simulink model "three_phase_dab"  (R2025b)
settings: Solver=ode23tb  StartTime=0.0  StopTime=simlength  FixedStep=tc  MaxStep=tc
values from neighbouring files (symbols this model uses):
  Idc_FS = max(Idab1_dc_nom,Idab2_dc_nom) * margin_factor    [init_model.m]
  tc = ts_dab/100    (= 4.16666666667e-07)    [init_model.m]
  Vdab2_dc_nom = 1500    [init_model.m]
  Vdc_FS = max(Vdab1_dc_nom,Vdab2_dc_nom) * margin_factor    [init_model.m]
libraries: fl_lib x27, nesl_utility x23, discrete_time_low_pass_filter x6, single_phase_transformer x3, single_phase_transformer_lib x3, litium_ion_battery x2, pi_ctrl x2, three_phase_inverter_ideal_switch_based_model x2, three_phase_inverter_mosfet_based_with_thermal_model x2, three_phase_dab_modulator x1
(part 1 of 2)
settings Model: SimulationMode=accelerator  Creator=LTNBDA  LastModifiedBy=dbagn
settings SolverCC: ZeroCrossControl=EnableAll  ZeroCrossAlgorithm=Adaptive  AlgebraicLoopSolver=TrustRegion  SolverResetMethod=Robust  AutoInsertRateTranBlk=on
settings DataIOCC: LimitDataPoints=on  MaxDataPoints=1  SaveFormat=Array  SignalLoggingSaveFormat=ModelDataLogs  SaveOutput=off  SignalLogging=off  DSMLogging=off  SaveTime=off  ReturnWorkspaceOutputs=off
settings OptimizationCC: ExpressionDepthLimit=2147483647.0  InitFltsAndDblsToZero=on  EfficientMapNaN2IntZero=off  LifeSpan=inf
settings DebuggingCC: SaveWithParameterizedLinksMsg=none  UnderspecifiedInitializationDetection=Classic  MergeDetectMultiDrivingBlocksExec=none  SignalResolutionControl=TryResolveAllWithWarning  SolverPrmCheckMsg=warning  MultiTaskDSMMsg=warning  MultiTaskCondExecSysMsg=none  MultiTaskRateTransMsg=warning  FcnCallInpInsideContextMsg=warning  StateNameClashWarn=warning  SFUnexpectedBacktrackingDiag=warning  SFNoUnconditionalDefaultTransitionDiag=warning  ArithmeticOperatorsInVariantConditions=warning
settings HardwareCC: ProdBitPerLong=64.0  ProdLargestAtomicFloat=None  ProdIntDivRoundTo=Undefined  ProdEndianess=Unspecified  ProdHWDeviceType=Generic->64-bit Embedded Processor (LP64)  TargetBitPerPointer=64.0  TargetBitPerSizeT=64.0  TargetBitPerPtrDiffT=64.0  TargetLongLongMode=on  TargetIntDivRoundTo=Zero  TargetEndianess=LittleEndian  TargetWordSize=64.0  TargetHWDeviceType=MATLAB Host  ProdEqTarget=off
settings ModelReferenceCC: EnableRefExpFcnMdlSchedulingChecks=on  PropagateSignalLabelsOutOfModel=off
settings SFSimCC: SimUseLocalCustomCode=off  CustomCodeUndefinedFunction=UseInterfaceOnly
settings RTWCC: RTWUseLocalCustomCode=off  GPUComputeCapability=3.5
settings CodeAppCC: MaxIdLength=128.0  StateflowObjectComments=on
settings GRTTargetCC: TargetLangStandard=C89/C90 (ANSI)  CombineOutputUpdateFcns=off  GRTInterface=on
settings ConfigComp: CovMetricSettings=dw  CovSaveCumulativeToWorkspaceVar=on  CovSaveSingleToWorkspaceVar=on  CovExternalEMLEnable=off
settings SimscapeCC: SimscapeNormalizeSystem=off

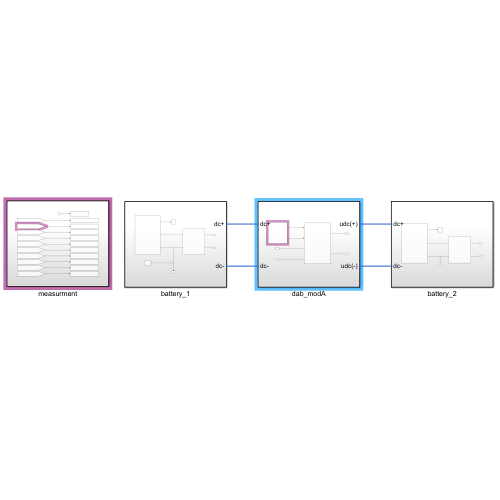
[thumbnail: Simulink's stored preview of the top-level diagram]
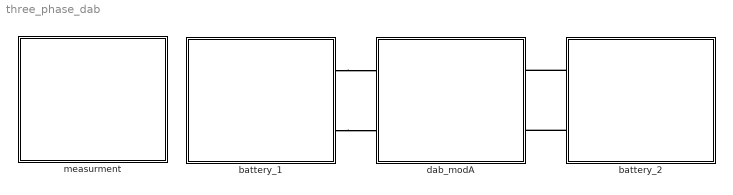
== system three_phase_dab ==
  battery_1 : Subsystem
  battery_2 : Subsystem
  dab_modA : Subsystem
  measurment : Subsystem
  connections:
  battery_2/RConn2 -- dab_modA/RConn2
  battery_2/RConn1 -- dab_modA/RConn1
  battery_1/RConn1 -- dab_modA/LConn1
  battery_1/RConn2 -- dab_modA/LConn2

== system three_phase_dab/battery_1 ==
  Electrical Reference1 : fl_lib/Electrical/Electrical Elements/Electrical Reference
  Solver Configuration : nesl_utility/Solver Configuration  PhysicalDomain=network_engine_domain  SubClassName=solver  LeftPortType=input  RightPortType=generic  Tones=[]  Harmonics=[]  SimulateNoise=off  Profile=off  UseLocalSampling=off  EnableSwitchedLinearOptims=on  FrequencyDomain=off  UseCCode=off  RelTol=0.001  AbsTol=0.001  MinStep=1e-09  ToWorkspace=off  RevertToSquareIcSolve=off  NumHomotopyIterations=100  PhasorMode=off  PhasorModeNumHarmonics=1  ConsistencySolver=NEWTON_FTOL  IndexReductionMethod=DerivativeReplacement  DoDC=off  ResidualTolerance=1e-09  ConsistencyTolSource=GLOBAL  ConsistencyAbsTol=0.001  ConsistencyRelTol=0.001  ConsistencyTolFactor=0.001  UseLocalSolver=on  LocalSolverChoice=NE_BACKWARD_EULER_ADVANCER  ResolveIndetEquations=on  FunctionEvalNumThread=1  LocalSolverSampleTime=tc  DoFixedCost=on  MaxNonlinIter=3  MaxModeIter=2  ComputeImpulses=off  ImpulseIterations=2  LinearAlgebra=auto  LinearAlgebraNumThread=0  EquationFormulation=NE_TIME_EF  DelaysMemoryBudget=1024  AutomaticFiltering=on  FilteringTimeConstant=0.001  PartitionStorageMethod=AS_NEEDED  PartitionMemoryBudget=1024  PartitionMethod=ROBUST  MultibodyUseLocalSolver=off  MultibodyLocalSolverChoice=ODE1  MultibodyLocalSolverSampleTime=0.001
  litium ion battery 1 : Scope
      settings: ActiveDisplayYMinimum=1095.5241232297076  ActiveDisplayYMaximum=1432.6160946881369  DataLoggingVariableName=ScopeData3
  litium_ion_battery : litium_ion_battery/litium_ion_battery  Q=50  number_of_cells=346  E_1=-1.031  E0=3.485  E1=0  E2=0  E3=0  Elog=-0.05  R0=0.035  R1=0.035  C1=0.5  M=125  alpha=35  soc_init=0.85  ts_battery=ts_battery  q1Kalman=q1Kalman  q2Kalman=q2Kalman  q3Kalman=q3Kalman  rKalman=rKalman  tc=tc
  single_phase_ui_measure : Subsystem
  dc+ : PMIOPort  Side=Right
  dc- : PMIOPort  Port=2  Side=Right
  wires:
  litium_ion_battery/1 -> litium ion battery 1/1
  connections:
  litium_ion_battery/RConn2 -- single_phase_ui_measure/LConn2 -- Electrical Reference1/LConn1 -- Solver Configuration/RConn1
  single_phase_ui_measure/RConn1 -- dc+/RConn1
  single_phase_ui_measure/LConn1 -- litium_ion_battery/RConn1
  dc-/RConn1 -- single_phase_ui_measure/RConn2

== system three_phase_dab/battery_2 ==
  Electrical Reference1 : fl_lib/Electrical/Electrical Elements/Electrical Reference
  litium ion battery 2 : Scope
      settings: ActiveDisplayYMinimum=-748.38980710578858  ActiveDisplayYMaximum=3166.4304287109808  DataLoggingVariableName=ScopeData3
  litium_ion_battery : litium_ion_battery/litium_ion_battery  Q=50  number_of_cells=346  E_1=-1.031  E0=3.485  E1=0  E2=0  E3=0  Elog=-0.05  R0=0.035  R1=0.035  C1=0.5  M=125  alpha=35  soc_init=0.85  ts_battery=ts_battery  q1Kalman=q1Kalman  q2Kalman=q2Kalman  q3Kalman=q3Kalman  rKalman=rKalman  tc=tc
  single_phase_ui_measure : Subsystem
  dc+ : PMIOPort  Side=Right
  dc- : PMIOPort  Port=2  Side=Right
  wires:
  litium_ion_battery/1 -> litium ion battery 2/1
  connections:
  dc-/RConn1 -- single_phase_ui_measure/RConn2
  single_phase_ui_measure/LConn1 -- litium_ion_battery/RConn1
  single_phase_ui_measure/RConn1 -- dc+/RConn1
  Electrical Reference1/LConn1 -- single_phase_ui_measure/LConn2 -- litium_ion_battery/RConn2

== system three_phase_dab/dab_modA ==
  dab_ctrl : Subsystem
  dcdc_with_galvanic_isolation : Subsystem
  udc(+) : PMIOPort  Side=Right
  udc(-) : PMIOPort  Port=2  Side=Right
  dc+ : PMIOPort  Port=3  Side=Left
  dc- : PMIOPort  Port=4  Side=Left
  wires:
  dab_ctrl/2(gate_commands_2) -> dcdc_with_galvanic_isolation/2(gate_commands_1)
  dab_ctrl/1(gate_commands_1) -> dcdc_with_galvanic_isolation/1(gate_commands_2)
  connections:
  udc(+)/RConn1 -- dcdc_with_galvanic_isolation/RConn1
  udc(-)/RConn1 -- dcdc_with_galvanic_isolation/RConn2
  dc-/RConn1 -- dcdc_with_galvanic_isolation/LConn2
  dc+/RConn1 -- dcdc_with_galvanic_isolation/LConn1

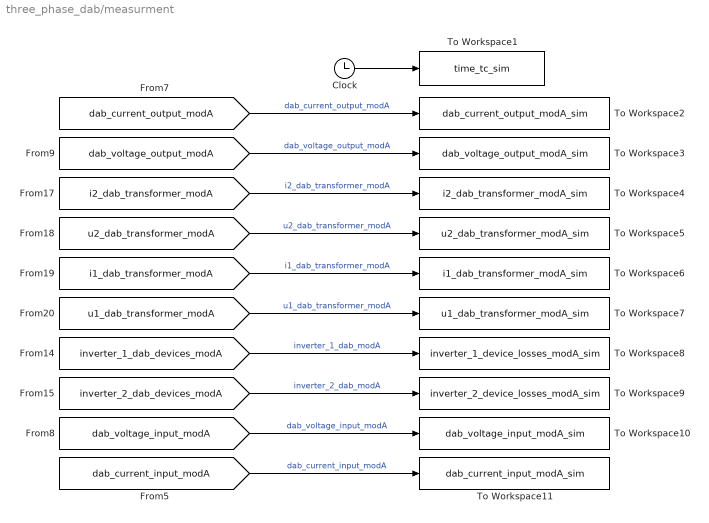
== system three_phase_dab/measurment ==
  Clock : Clock
  To Workspace1 : ToWorkspace  VariableName=time_tc_sim  SampleTime=tc
      settings: MaxDataPoints=Nc
  To Workspace10 : ToWorkspace  VariableName=dab_voltage_input_modA_sim  SampleTime=tc
      settings: MaxDataPoints=Nc
  To Workspace11 : ToWorkspace  VariableName=dab_current_input_modA_sim  SampleTime=tc
      settings: MaxDataPoints=Nc
  To Workspace2 : ToWorkspace  VariableName=dab_current_output_modA_sim  SampleTime=tc
      settings: MaxDataPoints=Nc
  To Workspace3 : ToWorkspace  VariableName=dab_voltage_output_modA_sim  SampleTime=tc
      settings: MaxDataPoints=Nc
  To Workspace4 : ToWorkspace  VariableName=i2_dab_transformer_modA_sim  SampleTime=tc
      settings: MaxDataPoints=Nc
  To Workspace5 : ToWorkspace  VariableName=u2_dab_transformer_modA_sim  SampleTime=tc
      settings: MaxDataPoints=Nc
  To Workspace6 : ToWorkspace  VariableName=i1_dab_transformer_modA_sim  SampleTime=tc
      settings: MaxDataPoints=Nc
  To Workspace7 : ToWorkspace  VariableName=u1_dab_transformer_modA_sim  SampleTime=tc
      settings: MaxDataPoints=Nc
  To Workspace8 : ToWorkspace  VariableName=inverter_1_device_losses_modA_sim  SampleTime=tc
      settings: MaxDataPoints=Nc
  To Workspace9 : ToWorkspace  VariableName=inverter_2_device_losses_modA_sim  SampleTime=tc
      settings: MaxDataPoints=Nc
  wires:
  Clock/1 -> To Workspace1/1
  [dab_current_output_modA] -> To Workspace2/1  "dab_current_output_modA"
  [dab_voltage_output_modA] -> To Workspace3/1  "dab_voltage_output_modA"
  [i2_dab_transformer_modA] -> To Workspace4/1  "i2_dab_transformer_modA"
  [u1_dab_transformer_modA] -> To Workspace7/1  "u1_dab_transformer_modA"
  [i1_dab_transformer_modA] -> To Workspace6/1  "i1_dab_transformer_modA"
  [u2_dab_transformer_modA] -> To Workspace5/1  "u2_dab_transformer_modA"
  [inverter_1_dab_devices_modA] -> To Workspace8/1  "inverter_1_dab_modA"
  [inverter_2_dab_devices_modA] -> To Workspace9/1  "inverter_2_dab_modA"
  [dab_voltage_input_modA] -> To Workspace10/1  "dab_voltage_input_modA"
  [dab_current_input_modA] -> To Workspace11/1  "dab_current_input_modA"

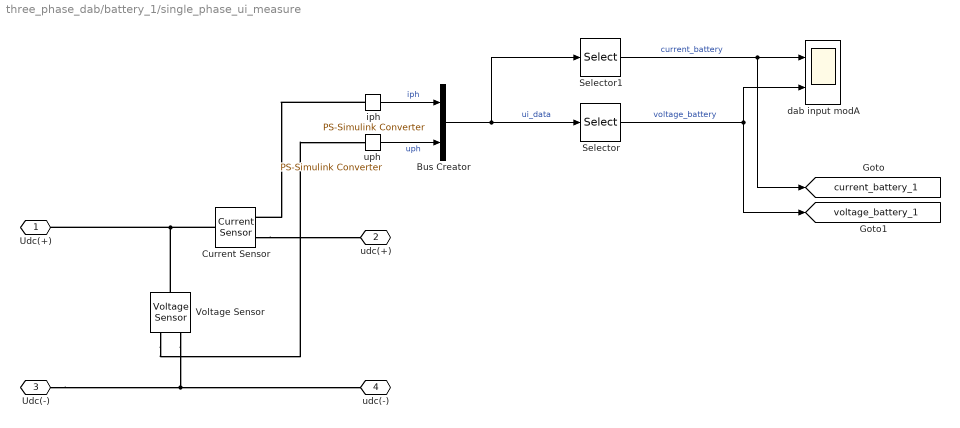
== system three_phase_dab/battery_1/single_phase_ui_measure ==
  Bus Creator : BusCreator  Inputs=2
  Current Sensor : fl_lib/Electrical/Electrical Sensors/Current Sensor
  Selector : Selector  InputPortWidth=2  IndexOptions=Index vector (dialog)  Indices=2  OutputSizes=1
  Selector1 : Selector  InputPortWidth=2  IndexOptions=Index vector (dialog)  Indices=1  OutputSizes=1
  Voltage Sensor : fl_lib/Electrical/Electrical Sensors/Voltage Sensor
  dab input modA : Scope  NumInputPorts=2
      settings: SampleTime=tc  ActiveDisplayYMinimum=-4428.9106738971032  ActiveDisplayYMaximum=4853.7975894934307  DataLoggingVariableName=ScopeData2
  iph : nesl_utility/PS-Simulink Converter  PhysicalDomain=network_engine_domain  SubClassName=ps_output  LeftPortType=input  RightPortType=output  PseudoPeriodic=off  Frequencies=[]  VectorFormat=1-D array  Unit=A  AffineConversion=off
  uph : nesl_utility/PS-Simulink Converter  PhysicalDomain=network_engine_domain  SubClassName=ps_output  LeftPortType=input  RightPortType=output  PseudoPeriodic=off  Frequencies=[]  VectorFormat=1-D array  Unit=V  AffineConversion=off
  Udc(+) : PMIOPort  Side=Left
  udc(+) : PMIOPort  Port=2  Side=Right
  Udc(-) : PMIOPort  Port=3  Side=Left
  udc(-) : PMIOPort  Port=4  Side=Right
  tag scope: current_battery_1=global, voltage_battery_1=global
  wires:
  Bus Creator/1 -> Selector/1, Selector1/1  "ui_data"
  iph/1 -> Bus Creator/1  "iph"
  uph/1 -> Bus Creator/2  "uph"
  Selector1/1 -> [current_battery_1], dab input modA/1  "current_battery"
  Selector/1 -> dab input modA/2, [voltage_battery_1]  "voltage_battery"
  connections:
  iph/LConn1 -- Current Sensor/RConn1
  Voltage Sensor/LConn1 -- Current Sensor/LConn1 -- Udc(+)/RConn1
  Current Sensor/RConn2 -- udc(+)/RConn1
  Voltage Sensor/RConn1 -- uph/LConn1
  Voltage Sensor/RConn2 -- Udc(-)/RConn1 -- udc(-)/RConn1

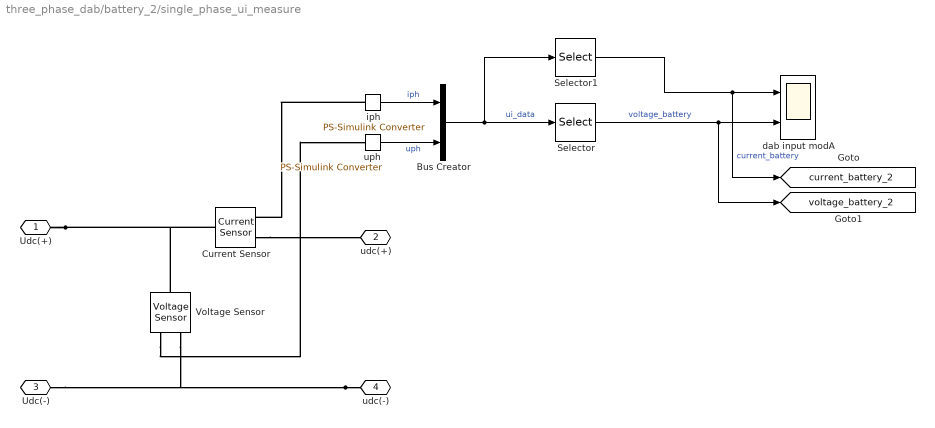
== system three_phase_dab/battery_2/single_phase_ui_measure ==
  Bus Creator : BusCreator  Inputs=2
  Current Sensor : fl_lib/Electrical/Electrical Sensors/Current Sensor
  Selector : Selector  InputPortWidth=2  IndexOptions=Index vector (dialog)  Indices=2  OutputSizes=1
  Selector1 : Selector  InputPortWidth=2  IndexOptions=Index vector (dialog)  Indices=1  OutputSizes=1
  Voltage Sensor : fl_lib/Electrical/Electrical Sensors/Voltage Sensor
  dab input modA : Scope  NumInputPorts=2
      settings: SampleTime=tc  ActiveDisplayYMinimum=-363.9315036867377  ActiveDisplayYMaximum=456.02820990604641  DataLoggingVariableName=ScopeData2
  iph : nesl_utility/PS-Simulink Converter  PhysicalDomain=network_engine_domain  SubClassName=ps_output  LeftPortType=input  RightPortType=output  PseudoPeriodic=off  Frequencies=[]  VectorFormat=1-D array  Unit=A  AffineConversion=off
  uph : nesl_utility/PS-Simulink Converter  PhysicalDomain=network_engine_domain  SubClassName=ps_output  LeftPortType=input  RightPortType=output  PseudoPeriodic=off  Frequencies=[]  VectorFormat=1-D array  Unit=V  AffineConversion=off
  Udc(+) : PMIOPort  Side=Left
  udc(+) : PMIOPort  Port=2  Side=Right
  Udc(-) : PMIOPort  Port=3  Side=Left
  udc(-) : PMIOPort  Port=4  Side=Right
  tag scope: current_battery_2=global, voltage_battery_2=global
  wires:
  Selector/1 -> [voltage_battery_2], dab input modA/2  "voltage_battery"
  Selector1/1 -> dab input modA/1, [current_battery_2]  "current_battery"
  uph/1 -> Bus Creator/2  "uph"
  iph/1 -> Bus Creator/1  "iph"
  Bus Creator/1 -> Selector1/1, Selector/1  "ui_data"
  connections:
  udc(-)/RConn1 -- Udc(-)/RConn1 -- Voltage Sensor/RConn2
  Voltage Sensor/RConn1 -- uph/LConn1
  Current Sensor/RConn2 -- udc(+)/RConn1
  Udc(+)/RConn1 -- Current Sensor/LConn1 -- Voltage Sensor/LConn1
  iph/LConn1 -- Current Sensor/RConn1

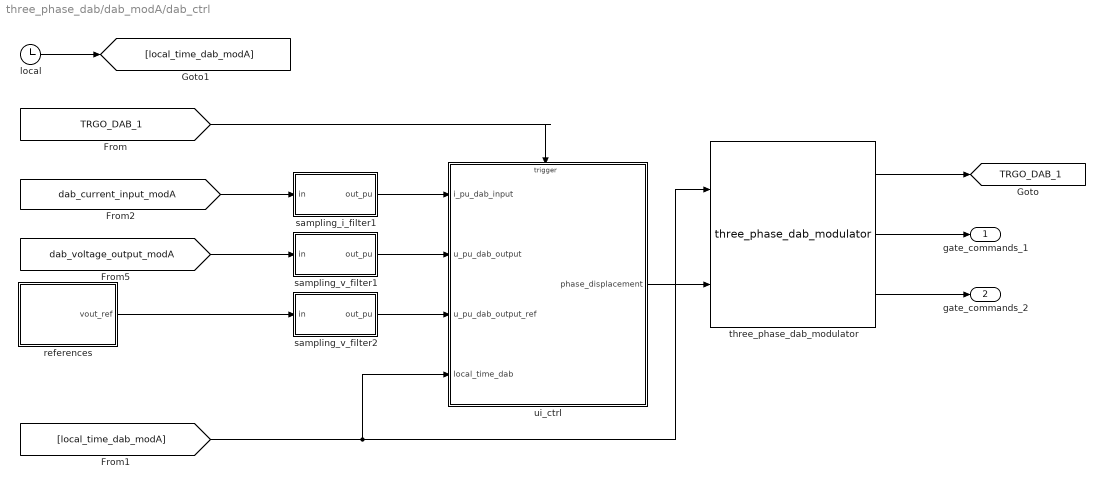
== system three_phase_dab/dab_modA/dab_ctrl ==
  local : Clock
  references : Subsystem
  sampling_i_filter1 : Subsystem
  sampling_v_filter1 : Subsystem
  sampling_v_filter2 : Subsystem
  three_phase_dab_modulator : three_phase_dab_modulator/three_phase_dab_modulator  fpwm=fPWM_DAB  tc=tc
  ui_ctrl : Subsystem
  gate_commands_1 : Outport
  gate_commands_2 : Outport  Port=2
  tag scope: TRGO_DAB_1=global
  wires:
  [dab_voltage_output_modA] -> sampling_v_filter1/1(in)
  [dab_current_input_modA] -> sampling_i_filter1/1(in)
  sampling_i_filter1/1(out_pu) -> ui_ctrl/1(i_pu_dab_input)
  sampling_v_filter1/1(out_pu) -> ui_ctrl/2(u_pu_dab_output)
  sampling_v_filter2/1(out_pu) -> ui_ctrl/3(u_pu_dab_output_ref)
  references/1(vout_ref) -> sampling_v_filter2/1(in)
  three_phase_dab_modulator/1 -> [TRGO_DAB_1]
  [TRGO_DAB_1] -> ui_ctrl/Trigger
  ui_ctrl/1(phase_displacement) -> three_phase_dab_modulator/2
  three_phase_dab_modulator/2 -> gate_commands_1/1
  three_phase_dab_modulator/3 -> gate_commands_2/1
  local/1 -> [local_time_dab_modA]
  [local_time_dab_modA] -> three_phase_dab_modulator/1, ui_ctrl/4(local_time_dab)

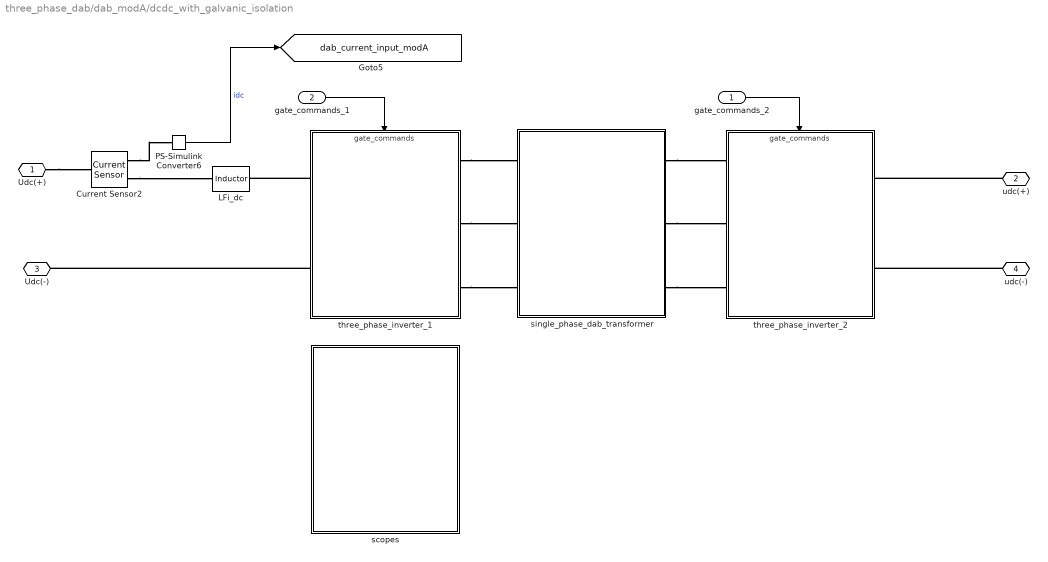
== system three_phase_dab/dab_modA/dcdc_with_galvanic_isolation ==
  gate_commands_2 : Inport
  gate_commands_1 : Inport  Port=2
  Current Sensor2 : fl_lib/Electrical/Electrical Sensors/Current Sensor
  LFi_dc : fl_lib/Electrical/Electrical Elements/Inductor  l=LFi_dc H  r=RLFi_dc Ohm  g=1e-9 1/Ohm  i_specify=off  i_priority=None  i=0 A  i_nominal_specify=off  i_nominal_value=1  i_nominal_unit=A  v_specify=off  v_priority=None  v=0 V  v_nominal_specify=off  v_nominal_value=1  v_nominal_unit=V  i_L_specify=off  i_L_priority=High  i_L=0 A  i_L_nominal_specify=off  i_L_nominal_value=1  i_L_nominal_unit=A
  PS-Simulink Converter6 : nesl_utility/PS-Simulink Converter  PhysicalDomain=network_engine_domain  SubClassName=ps_output  LeftPortType=input  RightPortType=output  PseudoPeriodic=off  Frequencies=[]  VectorFormat=1-D array  Unit=A  AffineConversion=on
  scopes : Subsystem
  single_phase_dab_transformer : Subsystem
  three_phase_inverter_1 : Subsystem
      settings: PortSchema="{\"entries\":[{\"content\":{\"sides\":[{\"content\":{\"connectorIds\":[\"LConn1\",\"LConn2\",\"LConn3\"]},\"type\":\"ConnectorPlacement.EquallySpacedRectSide\",\"uuid\":\"c872503a-61af-4937-bdf2-4de4f8645573\"},{\"content\":{\"connectorIds\":[\"RConn1\",\"RConn2\"],\"side\":\"RIGHT\"},\"type\":\"ConnectorPlacement.EquallySpacedRectSide\",\"uuid\":\"3b83f060-86a2-4569-84b5-d9f7c0485347\"},{\"content\":{\"connectorIds\":[\"In1\"],\"side\":\"TOP\"},\"type\":\"ConnectorPlacement.EquallySpacedRectSide\",\"uuid\":\"bf191d46-ce71-4d15-9dd0-24cc57253577\"}]},\"type\":\"ConnectorPlacement.EquallySpacedConnector\",\"uuid\":\"1b28ceee-25d0-45ae-a3c4-c2563f0d63ba\"}],\"packageUris\":[\"http://schema.mathworks.com/mf0/Connector/R2020b\"],\"version\":\"1.0\"}"
  three_phase_inverter_2 : Subsystem
      settings: PortSchema="{\"entries\":[{\"content\":{\"sides\":[{\"content\":{\"connectorIds\":[\"LConn1\",\"LConn2\",\"LConn3\"]},\"type\":\"ConnectorPlacement.EquallySpacedRectSide\",\"uuid\":\"c872503a-61af-4937-bdf2-4de4f8645573\"},{\"content\":{\"connectorIds\":[\"RConn1\",\"RConn2\"],\"side\":\"RIGHT\"},\"type\":\"ConnectorPlacement.EquallySpacedRectSide\",\"uuid\":\"3b83f060-86a2-4569-84b5-d9f7c0485347\"},{\"content\":{\"connectorIds\":[\"In1\"],\"side\":\"TOP\"},\"type\":\"ConnectorPlacement.EquallySpacedRectSide\",\"uuid\":\"bf191d46-ce71-4d15-9dd0-24cc57253577\"}]},\"type\":\"ConnectorPlacement.EquallySpacedConnector\",\"uuid\":\"1b28ceee-25d0-45ae-a3c4-c2563f0d63ba\"}],\"packageUris\":[\"http://schema.mathworks.com/mf0/Connector/R2020b\"],\"version\":\"1.0\"}"
  Udc(+) : PMIOPort  Side=Left
  udc(+) : PMIOPort  Port=2  Side=Right
  Udc(-) : PMIOPort  Port=3  Side=Left
  udc(-) : PMIOPort  Port=4  Side=Right
  tag scope: dab_current_input_modA=global
  wires:
  PS-Simulink Converter6/1 -> [dab_current_input_modA]  "idc"
  gate_commands_1/1 -> three_phase_inverter_1/1(gate_commands)
  gate_commands_2/1 -> three_phase_inverter_2/1(gate_commands)
  connections:
  three_phase_inverter_1/RConn1 -- LFi_dc/RConn1
  three_phase_inverter_1/RConn2 -- Udc(-)/RConn1
  udc(-)/RConn1 -- three_phase_inverter_2/RConn2
  Current Sensor2/RConn2 -- LFi_dc/LConn1
  Udc(+)/RConn1 -- Current Sensor2/LConn1
  Current Sensor2/RConn1 -- PS-Simulink Converter6/LConn1
  udc(+)/RConn1 -- three_phase_inverter_2/RConn1
  three_phase_inverter_1/LConn1 -- single_phase_dab_transformer/LConn1
  three_phase_inverter_1/LConn2 -- single_phase_dab_transformer/LConn2
  three_phase_inverter_1/LConn3 -- single_phase_dab_transformer/LConn3
  single_phase_dab_transformer/RConn1 -- three_phase_inverter_2/LConn1
  single_phase_dab_transformer/RConn2 -- three_phase_inverter_2/LConn2
  single_phase_dab_transformer/RConn3 -- three_phase_inverter_2/LConn3

== system three_phase_dab/dab_modA/dab_ctrl/references ==
  Rate Limiter : RateLimiter  RisingSlewLimit=Vdab2_dc_nom*10  FallingSlewLimit=-Vdab2_dc_nom*10  SampleTimeMode=inherited
  Vout_dc_nom : Step  Time=1e-3  After=Vdab2_dc_nom  SampleTime=0
  vout_ref : Outport
  wires:
  Rate Limiter/1 -> vout_ref/1
  Vout_dc_nom/1 -> Rate Limiter/1

== system three_phase_dab/dab_modA/dab_ctrl/sampling_i_filter1 ==
  in : Inport
  1/Ti3 : Gain  Gain=1/Idc_FS  OutDataTypeStr=double  SaturateOnIntegerOverflow=on  ParamDataTypeStr=Inherit: Same as input
  out_pu : Outport
  wires:
  in/1 -> 1/Ti3/1
  1/Ti3/1 -> out_pu/1

== system three_phase_dab/dab_modA/dab_ctrl/sampling_v_filter1 ==
  in : Inport
  1/Ti3 : Gain  Gain=1/Vdc_FS  OutDataTypeStr=double  SaturateOnIntegerOverflow=on  ParamDataTypeStr=Inherit: Same as input
  out_pu : Outport
  wires:
  in/1 -> 1/Ti3/1
  1/Ti3/1 -> out_pu/1

== system three_phase_dab/dab_modA/dab_ctrl/sampling_v_filter2 ==
  in : Inport
  1/Ti3 : Gain  Gain=1/Vdc_FS  OutDataTypeStr=double  SaturateOnIntegerOverflow=on  ParamDataTypeStr=Inherit: Same as input
  Saturation : Saturate  UpperLimit=1  LowerLimit=0  OutDataTypeStr=double
  out_pu : Outport
  wires:
  in/1 -> 1/Ti3/1
  1/Ti3/1 -> Saturation/1
  Saturation/1 -> out_pu/1

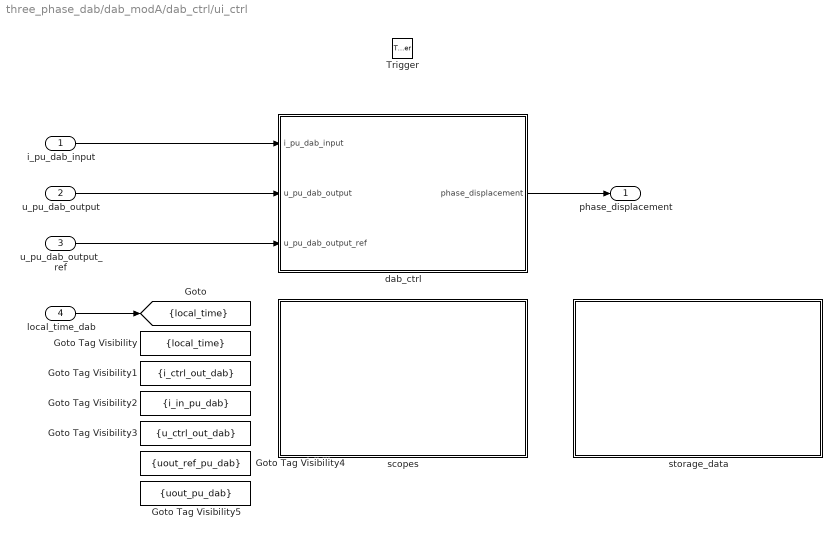
== system three_phase_dab/dab_modA/dab_ctrl/ui_ctrl ==
  i_pu_dab_input : Inport
  u_pu_dab_output : Inport  Port=2
  u_pu_dab_output_ref : Inport  Port=3
  local_time_dab : Inport  Port=4
  Trigger : TriggerPort  VariantControl=(inherit)  PortDimensions=1
  Goto Tag Visibility : GotoTagVisibility  GotoTag=local_time
  Goto Tag Visibility1 : GotoTagVisibility  GotoTag=i_ctrl_out_dab
  Goto Tag Visibility2 : GotoTagVisibility  GotoTag=i_in_pu_dab
  Goto Tag Visibility3 : GotoTagVisibility  GotoTag=u_ctrl_out_dab
  Goto Tag Visibility4 : GotoTagVisibility  GotoTag=uout_ref_pu_dab
  Goto Tag Visibility5 : GotoTagVisibility  GotoTag=uout_pu_dab
  dab_ctrl : Subsystem
  scopes : Subsystem
  storage_data : Subsystem
  phase_displacement : Outport
  tag scope: local_time=scoped
  wires:
  i_pu_dab_input/1 -> dab_ctrl/1(i_pu_dab_input)
  u_pu_dab_output/1 -> dab_ctrl/2(u_pu_dab_output)
  u_pu_dab_output_ref/1 -> dab_ctrl/3(u_pu_dab_output_ref)
  dab_ctrl/1(phase_displacement) -> phase_displacement/1
  local_time_dab/1 -> [local_time]

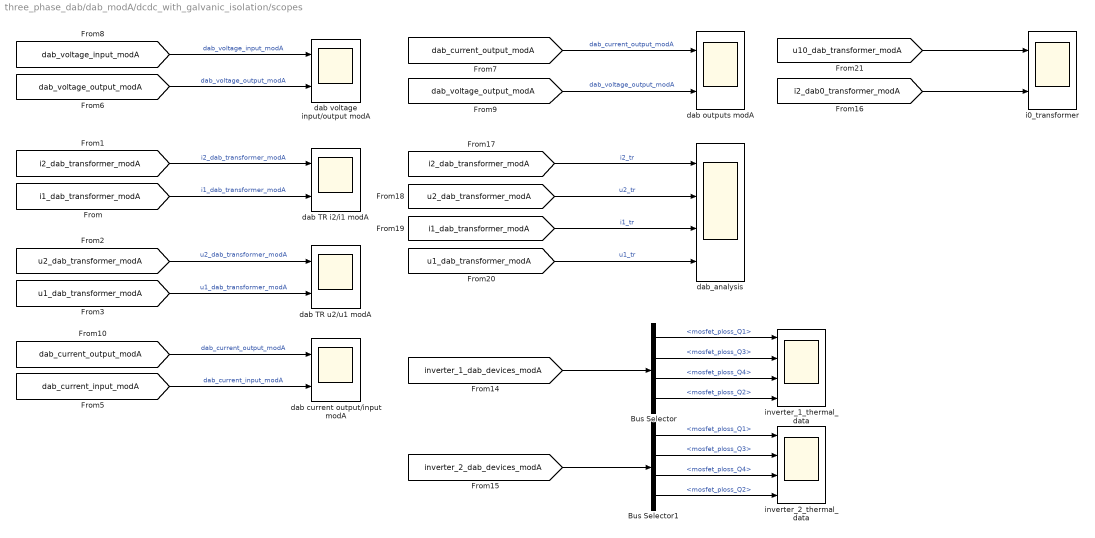
== system three_phase_dab/dab_modA/dcdc_with_galvanic_isolation/scopes ==
  Bus Selector : BusSelector  OutputSignals=mosfet_ploss_Q1,mosfet_ploss_Q3,mosfet_ploss_Q4,mosfet_ploss_Q2
  Bus Selector1 : BusSelector  OutputSignals=mosfet_ploss_Q1,mosfet_ploss_Q3,mosfet_ploss_Q4,mosfet_ploss_Q2
  dab TR i2/i1 modA : Scope  NumInputPorts=2
      settings: SampleTime=tc  ActiveDisplayYMinimum=-769.76570927697639  ActiveDisplayYMaximum=617.34679539784429  DataLoggingVariableName=ScopeData13
  dab TR u2/u1 modA : Scope  NumInputPorts=2
      settings: SampleTime=tc  ActiveDisplayYMinimum=-1578.7453878307324  ActiveDisplayYMaximum=1578.7340154658184  DataLoggingVariableName=ScopeData4
  dab current output/input modA : Scope  NumInputPorts=2
      settings: SampleTime=tc  ActiveDisplayYMinimum=-410.50779379600635  ActiveDisplayYMaximum=588.57119970360964  DataLoggingVariableName=ScopeData8
  dab outputs modA : Scope  NumInputPorts=2
      settings: SampleTime=tc  ActiveDisplayYMinimum=-911.87281827356537  ActiveDisplayYMaximum=678.26507696890121  DataLoggingVariableName=ScopeData6
  dab voltage input/output modA : Scope  NumInputPorts=2
      settings: SampleTime=tc  ActiveDisplayYMinimum=1151.9301233458582  ActiveDisplayYMaximum=1294.7889710686802  DataLoggingVariableName=ScopeData10
  dab_analysis : Scope  NumInputPorts=4
      settings: SampleTime=tc  ActiveDisplayYMinimum=-2819.8939411691067  ActiveDisplayYMaximum=1653.00985583068  DataLoggingVariableName=ScopeData14
  i0_transformer : Scope  NumInputPorts=2
      settings: SampleTime=tc  ActiveDisplayYMinimum=-1.8947806286936003E-13  ActiveDisplayYMaximum=1.8947806286936003E-13  DataLoggingVariableName=ScopeData11
  inverter_1_thermal_data : Scope  NumInputPorts=4
      settings: SampleTime=tc  ActiveDisplayYMinimum=-41.628226428892724  ActiveDisplayYMaximum=374.65403786003458
  inverter_2_thermal_data : Scope  NumInputPorts=4
      settings: SampleTime=tc  ActiveDisplayYMinimum=-51.964921296072347  ActiveDisplayYMaximum=467.68429166465125  DataLoggingVariableName=ScopeData9
  wires:
  [dab_voltage_input_modA] -> dab voltage input/output modA/1  "dab_voltage_input_modA"
  [dab_current_output_modA] -> dab current output/input modA/1  "dab_current_output_modA"
  [dab_voltage_output_modA] -> dab voltage input/output modA/2  "dab_voltage_output_modA"
  [dab_current_input_modA] -> dab current output/input modA/2  "dab_current_input_modA"
  [i2_dab_transformer_modA] -> dab TR i2/i1 modA/1  "i2_dab_transformer_modA"
  [i1_dab_transformer_modA] -> dab TR i2/i1 modA/2  "i1_dab_transformer_modA"
  [u2_dab_transformer_modA] -> dab TR u2/u1 modA/1  "u2_dab_transformer_modA"
  [u1_dab_transformer_modA] -> dab TR u2/u1 modA/2  "u1_dab_transformer_modA"
  [dab_voltage_output_modA] -> dab outputs modA/2  "dab_voltage_output_modA"
  [dab_current_output_modA] -> dab outputs modA/1  "dab_current_output_modA"
  [inverter_1_dab_devices_modA] -> Bus Selector/1
  Bus Selector/1 -> inverter_1_thermal_data/1  "<mosfet_ploss_Q1>"
  Bus Selector/2 -> inverter_1_thermal_data/2  "<mosfet_ploss_Q3>"
  Bus Selector/3 -> inverter_1_thermal_data/3  "<mosfet_ploss_Q4>"
  Bus Selector/4 -> inverter_1_thermal_data/4  "<mosfet_ploss_Q2>"
  Bus Selector1/4 -> inverter_2_thermal_data/4  "<mosfet_ploss_Q2>"
  Bus Selector1/3 -> inverter_2_thermal_data/3  "<mosfet_ploss_Q4>"
  Bus Selector1/2 -> inverter_2_thermal_data/2  "<mosfet_ploss_Q3>"
  Bus Selector1/1 -> inverter_2_thermal_data/1  "<mosfet_ploss_Q1>"
  [inverter_2_dab_devices_modA] -> Bus Selector1/1
  [i2_dab0_transformer_modA] -> i0_transformer/2
  [u10_dab_transformer_modA] -> i0_transformer/1
  [u2_dab_transformer_modA] -> dab_analysis/2  "u2_tr"
  [i2_dab_transformer_modA] -> dab_analysis/1  "i2_tr"
  [u1_dab_transformer_modA] -> dab_analysis/4  "u1_tr"
  [i1_dab_transformer_modA] -> dab_analysis/3  "i1_tr"

== system three_phase_dab/dab_modA/dcdc_with_galvanic_isolation/single_phase_dab_transformer ==
  three_phase_hf_transformer : Subsystem
  three_phase_hf_transformer1 : Subsystem  Commented=on
  threephase_vi_measures_stack : Subsystem
  threephase_vi_measures_stack1 : Subsystem
  u1 : PMIOPort  Side=Left
  v1 : PMIOPort  Port=2  Side=Left
  w1 : PMIOPort  Port=3  Side=Left
  u2 : PMIOPort  Port=4  Side=Right
  v2 : PMIOPort  Port=5  Side=Right
  w2 : PMIOPort  Port=6  Side=Right
  connections:
  three_phase_hf_transformer/LConn1 -- threephase_vi_measures_stack/RConn1
  three_phase_hf_transformer/LConn2 -- threephase_vi_measures_stack/RConn2
  three_phase_hf_transformer/LConn3 -- threephase_vi_measures_stack/RConn3
  threephase_vi_measures_stack1/LConn1 -- three_phase_hf_transformer/RConn1
  threephase_vi_measures_stack1/LConn2 -- three_phase_hf_transformer/RConn2
  threephase_vi_measures_stack1/LConn3 -- three_phase_hf_transformer/RConn3
  threephase_vi_measures_stack1/LConn4 -- three_phase_hf_transformer/RConn4
  threephase_vi_measures_stack/RConn4 -- three_phase_hf_transformer/LConn4
  u1/RConn1 -- threephase_vi_measures_stack/LConn1
  v1/RConn1 -- threephase_vi_measures_stack/LConn2
  w1/RConn1 -- threephase_vi_measures_stack/LConn3
  v2/RConn1 -- threephase_vi_measures_stack1/RConn2
  w2/RConn1 -- threephase_vi_measures_stack1/RConn3
  threephase_vi_measures_stack1/RConn1 -- u2/RConn1

== system three_phase_dab/dab_modA/dcdc_with_galvanic_isolation/three_phase_inverter_1 ==
  gate_commands : Inport
  dclink_1 : Subsystem
  three_phase_inverter_1 : Subsystem
  u : PMIOPort  Side=Left
  v : PMIOPort  Port=2  Side=Left
  Udc(+) : PMIOPort  Port=3  Side=Right
  Udc(-) : PMIOPort  Port=4  Side=Right
  w : PMIOPort  Port=5  Side=Left
  wires:
  gate_commands/1 -> three_phase_inverter_1/1(gate_commands)
  connections:
  Udc(+)/RConn1 -- dclink_1/LConn1
  Udc(-)/RConn1 -- dclink_1/LConn2
  dclink_1/RConn1 -- three_phase_inverter_1/LConn1
  three_phase_inverter_1/RConn1 -- u/RConn1
  three_phase_inverter_1/RConn2 -- v/RConn1
  three_phase_inverter_1/LConn2 -- dclink_1/RConn2
  w/RConn1 -- three_phase_inverter_1/RConn3

== system three_phase_dab/dab_modA/dcdc_with_galvanic_isolation/three_phase_inverter_2 ==
  gate_commands : Inport
  dclink_2 : Subsystem
  three_phase_inverter_2 : Subsystem
  u : PMIOPort  Side=Left
  v : PMIOPort  Port=2  Side=Left
  udc(+) : PMIOPort  Port=3  Side=Right
  udc(-) : PMIOPort  Port=4  Side=Right
  w : PMIOPort  Port=5  Side=Left
  wires:
  gate_commands/1 -> three_phase_inverter_2/1(gate_commands)
  connections:
  udc(+)/RConn1 -- dclink_2/RConn1
  udc(-)/RConn1 -- dclink_2/RConn2
  dclink_2/LConn1 -- three_phase_inverter_2/RConn1
  u/RConn1 -- three_phase_inverter_2/LConn1
  v/RConn1 -- three_phase_inverter_2/LConn2
  dclink_2/LConn2 -- three_phase_inverter_2/RConn2
  w/RConn1 -- three_phase_inverter_2/LConn3

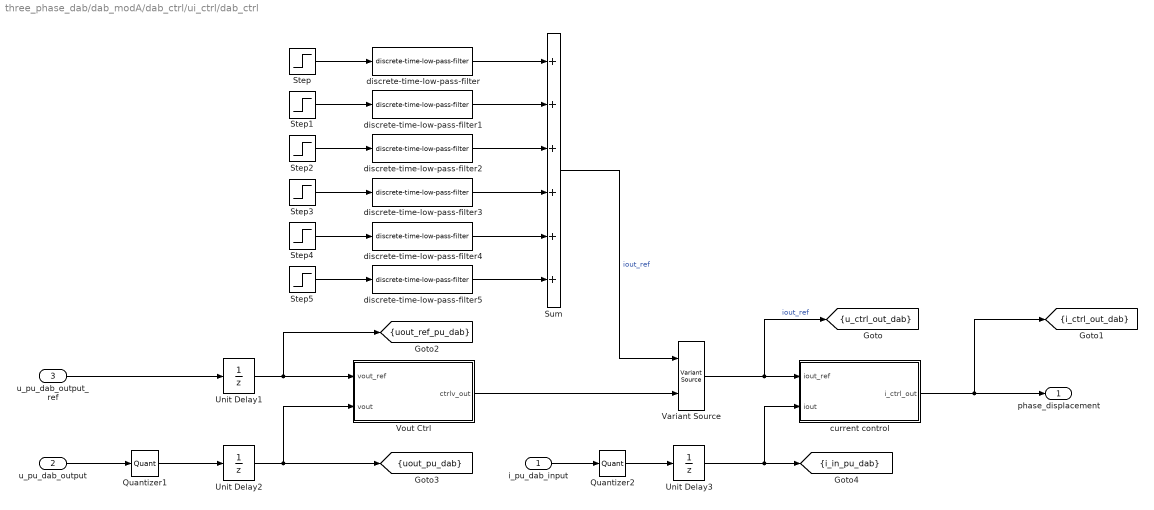
== system three_phase_dab/dab_modA/dab_ctrl/ui_ctrl/dab_ctrl ==
  i_pu_dab_input : Inport
  u_pu_dab_output : Inport  Port=2
  u_pu_dab_output_ref : Inport  Port=3
  Quantizer1 : Quantizer  QuantizationInterval=adc12_quantization
  Quantizer2 : Quantizer  QuantizationInterval=adc12_quantization
  Step : Step  Time=0.05  After=0.25
  Step1 : Step  Time=0.4  After=0.75
  Step2 : Step  Time=0.6  After=0.25
  Step3 : Step  Time=0.8  After=-1
  Step4 : Step  After=-0.75
  Step5 : Step  Time=1.25  After=-0.5
  Sum : Sum  Inputs=++++++
  Unit Delay1 : UnitDelay  SampleTime=-1  HasFrameUpgradeWarning=on
  Unit Delay2 : UnitDelay  SampleTime=-1  HasFrameUpgradeWarning=on
  Unit Delay3 : UnitDelay  SampleTime=-1  HasFrameUpgradeWarning=on
  Variant Source : VariantSource  VariantControls={true, false}
  Vout Ctrl : Subsystem
  current control : Subsystem
  discrete-time-low-pass-filter{,1..5} (6 alike) : discrete_time_low_pass_filter/discrete-time-low-pass-filter  tau=0.02  ts=ts_dab
  phase_displacement : Outport
  tag scope: i_ctrl_out_dab=scoped, i_in_pu_dab=scoped, u_ctrl_out_dab=scoped, uout_pu_dab=scoped, uout_ref_pu_dab=scoped
  wires:
  Vout Ctrl/1(ctrlv_out) -> Variant Source/2
  Variant Source/1 -> [u_ctrl_out_dab], current control/1(iout_ref)  "iout_ref"
  i_pu_dab_input/1 -> Quantizer2/1
  Sum/1 -> Variant Source/1  "iout_ref"
  current control/1(i_ctrl_out) -> phase_displacement/1, [i_ctrl_out_dab]
  Unit Delay3/1 -> current control/2(iout), [i_in_pu_dab]
  Unit Delay2/1 -> [uout_pu_dab], Vout Ctrl/2(vout)
  Unit Delay1/1 -> Vout Ctrl/1(vout_ref), [uout_ref_pu_dab]
  u_pu_dab_output/1 -> Quantizer1/1
  Step/1 -> discrete-time-low-pass-filter/1
  Step1/1 -> discrete-time-low-pass-filter1/1
  Step2/1 -> discrete-time-low-pass-filter2/1
  Step3/1 -> discrete-time-low-pass-filter3/1
  Step4/1 -> discrete-time-low-pass-filter4/1
  Step5/1 -> discrete-time-low-pass-filter5/1
  discrete-time-low-pass-filter/1 -> Sum/1
  discrete-time-low-pass-filter1/1 -> Sum/2
  discrete-time-low-pass-filter2/1 -> Sum/3
  discrete-time-low-pass-filter3/1 -> Sum/4
  discrete-time-low-pass-filter4/1 -> Sum/5
  discrete-time-low-pass-filter5/1 -> Sum/6
  u_pu_dab_output_ref/1 -> Unit Delay1/1
  Quantizer1/1 -> Unit Delay2/1
  Quantizer2/1 -> Unit Delay3/1

== system three_phase_dab/dab_modA/dab_ctrl/ui_ctrl/scopes ==
  Bus Creator : BusCreator  Inputs=2
  Bus Creator1 : BusCreator  Inputs=2
  dab-tracking : Scope  NumInputPorts=2
      settings: ActiveDisplayYMinimum=-2.3268130293516371  ActiveDisplayYMaximum=3.0115670177424061  DataLoggingVariableName=ScopeData7
  u_ctrl_out_dab/i_ctrl_out_dab : Scope  NumInputPorts=2
      settings: ActiveDisplayYMinimum=-1.2812486231311795  ActiveDisplayYMaximum=1.531237608180616
  wires:
  Bus Creator1/1 -> dab-tracking/2
  Bus Creator/1 -> dab-tracking/1
  [i_ctrl_out_dab] -> u_ctrl_out_dab/i_ctrl_out_dab/2  "i_ctrl_out_dab"
  [i_in_pu_dab] -> Bus Creator1/2  "i_in_pu_dab"
  [uout_ref_pu_dab] -> Bus Creator/1  "uout_ref_pu_dab"
  [u_ctrl_out_dab] -> u_ctrl_out_dab/i_ctrl_out_dab/1  "u_ctrl_out_dab"
  [u_ctrl_out_dab] -> Bus Creator1/1  "u_ctrl_out_dab"
  [uout_pu_dab] -> Bus Creator/2  "uout_pu_dab"

== system three_phase_dab/dab_modA/dab_ctrl/ui_ctrl/storage_data ==
  To Workspace1 : ToWorkspace  VariableName=time_ts_dab_sim  SampleTime=-1
      settings: MaxDataPoints=Ns_dab
  To Workspace2 : ToWorkspace  VariableName=i_in_pu_dab_modA_sim  SampleTime=-1
      settings: MaxDataPoints=Ns_dab
  To Workspace3 : ToWorkspace  VariableName=i_in_pu_ref_dab_modA_sim  SampleTime=-1
      settings: MaxDataPoints=Ns_dab
  To Workspace4 : ToWorkspace  VariableName=i_ctrl_out_dab_modA_sim  SampleTime=-1
      settings: MaxDataPoints=Ns_dab
  wires:
  [u_ctrl_out_dab] -> To Workspace3/1  "u_ctrl_out_dab"
  [i_ctrl_out_dab] -> To Workspace4/1  "i_ctrl_out_dab"
  [i_in_pu_dab] -> To Workspace2/1  "i_in_pu_dab"
  [local_time] -> To Workspace1/1  "local_time"

== system three_phase_dab/dab_modA/dcdc_with_galvanic_isolation/single_phase_dab_transformer/three_phase_hf_transformer ==
  single_phase_transformer_1 : single_phase_transformer/single_phase_transformer  lm_trafo=lm_trafo  m1=m1  m2=m2  rd1_trafo=rd1_trafo  rd2_trafo=rd2_trafo  ld1_trafo=ld1_trafo  ld2_trafo=ld2_trafo  rfe_trafo=rfe_trafo  length_core=1  mu0=1.256637e-6  mur=10e3
  single_phase_transformer_2 : single_phase_transformer/single_phase_transformer  lm_trafo=lm_trafo  m1=m1  m2=m2  rd1_trafo=rd1_trafo  rd2_trafo=rd2_trafo  ld1_trafo=ld1_trafo  ld2_trafo=ld2_trafo  rfe_trafo=rfe_trafo  length_core=1  mu0=1.256637e-6  mur=10e3
  single_phase_transformer_2: data : Scope
      settings: ActiveDisplayYMinimum=-1744.0416508829171  ActiveDisplayYMaximum=1756.9104494327478  DataLoggingVariableName=ScopeData15
  single_phase_transformer_3 : single_phase_transformer/single_phase_transformer  lm_trafo=lm_trafo  m1=m1  m2=m2  rd1_trafo=rd1_trafo  rd2_trafo=rd2_trafo  ld1_trafo=ld1_trafo  ld2_trafo=ld2_trafo  rfe_trafo=rfe_trafo  length_core=1  mu0=1.256637e-6  mur=10e3
  ua1 : PMIOPort  Side=Left
  ua2 : PMIOPort  Port=2  Side=Right
  ub1 : PMIOPort  Port=3  Side=Left
  ub2 : PMIOPort  Port=4  Side=Right
  uc1 : PMIOPort  Port=5  Side=Left
  uc2 : PMIOPort  Port=6  Side=Right
  un1 : PMIOPort  Port=7  Side=Left
  un2 : PMIOPort  Port=8  Side=Right
  wires:
  single_phase_transformer_2/1 -> single_phase_transformer_2: data/1
  connections:
  un2/RConn1 -- single_phase_transformer_2/RConn2 -- single_phase_transformer_1/RConn2 -- single_phase_transformer_3/RConn2
  un1/RConn1 -- single_phase_transformer_2/LConn2 -- single_phase_transformer_1/LConn2 -- single_phase_transformer_3/LConn2
  single_phase_transformer_1/LConn1 -- ua1/RConn1
  single_phase_transformer_2/LConn1 -- ub1/RConn1
  single_phase_transformer_3/LConn1 -- uc1/RConn1
  single_phase_transformer_3/RConn1 -- uc2/RConn1
  single_phase_transformer_2/RConn1 -- ub2/RConn1
  single_phase_transformer_1/RConn1 -- ua2/RConn1

== system three_phase_dab/dab_modA/dcdc_with_galvanic_isolation/single_phase_dab_transformer/three_phase_hf_transformer1 ==
  tr1 : single_phase_transformer_lib/single phase transformer  Lm=lm_trafo H  n1=m1  n2=m2  Rd1=rd1_trafo Ohm  Rd2=rd2_trafo Ohm  Ld1=ld1_trafo H  Ld2=ld2_trafo H  Rfe=rfe_trafo Ohm  phi_specify=off  phi_priority=None  phi=0 V*s  phi_nominal_specify=off  phi_nominal_value=1  phi_nominal_unit=V*s  i1_specify=on  i1_priority=High  i1=0 A  i1_nominal_specify=off  i1_nominal_value=1  i1_nominal_unit=A  i2_specify=on  i2_priority=High  i2=0 A  i2_nominal_specify=off  i2_nominal_value=1  i2_nominal_unit=A  ife_specify=off  ife_priority=None  ife=0 A  ife_nominal_specify=off  ife_nominal_value=1  ife_nominal_unit=A  u1_specify=off  u1_priority=None  u1=0 V  u1_nominal_specify=off  u1_nominal_value=1  u1_nominal_unit=V  u2_specify=off  u2_priority=None  u2=0 V  u2_nominal_specify=off  u2_nominal_value=1  u2_nominal_unit=V
      settings: InternalSimscapePortConfiguration="{\"Bottom\":[],\"Left\":[{\"id\":\"u1_p\",\"label\":\"u1(+)\",\"type\":\"foundation.electrical.electrical\"},{\"id\":\"u1_n\",\"label\":\"u1(-)\",\"type\":\"foundation.electrical.electrical\"}],\"Right\":[{\"id\":\"u2_p\",\"label\":\"u2(+)\",\"type\":\"foundation.electrical.electrical\"},{\"id\":\"u2_n\",\"label\":\"u2(-)\",\"type\":\"foundation.electrical.electrical\"}],\"Top\":[]}"
  tr2 : single_phase_transformer_lib/single phase transformer  Lm=lm_trafo H  n1=m1  n2=m2  Rd1=rd1_trafo Ohm  Rd2=rd2_trafo Ohm  Ld1=ld1_trafo H  Ld2=ld2_trafo H  Rfe=rfe_trafo Ohm  phi_specify=off  phi_priority=None  phi=0 V*s  phi_nominal_specify=off  phi_nominal_value=1  phi_nominal_unit=V*s  i1_specify=on  i1_priority=High  i1=0 A  i1_nominal_specify=off  i1_nominal_value=1  i1_nominal_unit=A  i2_specify=on  i2_priority=High  i2=0 A  i2_nominal_specify=off  i2_nominal_value=1  i2_nominal_unit=A  ife_specify=off  ife_priority=None  ife=0 A  ife_nominal_specify=off  ife_nominal_value=1  ife_nominal_unit=A  u1_specify=off  u1_priority=None  u1=0 V  u1_nominal_specify=off  u1_nominal_value=1  u1_nominal_unit=V  u2_specify=off  u2_priority=None  u2=0 V  u2_nominal_specify=off  u2_nominal_value=1  u2_nominal_unit=V
      settings: InternalSimscapePortConfiguration="{\"Bottom\":[],\"Left\":[{\"id\":\"u1_p\",\"label\":\"u1(+)\",\"type\":\"foundation.electrical.electrical\"},{\"id\":\"u1_n\",\"label\":\"u1(-)\",\"type\":\"foundation.electrical.electrical\"}],\"Right\":[{\"id\":\"u2_p\",\"label\":\"u2(+)\",\"type\":\"foundation.electrical.electrical\"},{\"id\":\"u2_n\",\"label\":\"u2(-)\",\"type\":\"foundation.electrical.electrical\"}],\"Top\":[]}"
  tr3 : single_phase_transformer_lib/single phase transformer  Lm=lm_trafo H  n1=m1  n2=m2  Rd1=rd1_trafo Ohm  Rd2=rd2_trafo Ohm  Ld1=ld1_trafo H  Ld2=ld2_trafo H  Rfe=rfe_trafo Ohm  phi_specify=off  phi_priority=None  phi=0 V*s  phi_nominal_specify=off  phi_nominal_value=1  phi_nominal_unit=V*s  i1_specify=on  i1_priority=High  i1=0 A  i1_nominal_specify=off  i1_nominal_value=1  i1_nominal_unit=A  i2_specify=on  i2_priority=High  i2=0 A  i2_nominal_specify=off  i2_nominal_value=1  i2_nominal_unit=A  ife_specify=off  ife_priority=None  ife=0 A  ife_nominal_specify=off  ife_nominal_value=1  ife_nominal_unit=A  u1_specify=off  u1_priority=None  u1=0 V  u1_nominal_specify=off  u1_nominal_value=1  u1_nominal_unit=V  u2_specify=off  u2_priority=None  u2=0 V  u2_nominal_specify=off  u2_nominal_value=1  u2_nominal_unit=V
      settings: InternalSimscapePortConfiguration="{\"Bottom\":[],\"Left\":[{\"id\":\"u1_p\",\"label\":\"u1(+)\",\"type\":\"foundation.electrical.electrical\"},{\"id\":\"u1_n\",\"label\":\"u1(-)\",\"type\":\"foundation.electrical.electrical\"}],\"Right\":[{\"id\":\"u2_p\",\"label\":\"u2(+)\",\"type\":\"foundation.electrical.electrical\"},{\"id\":\"u2_n\",\"label\":\"u2(-)\",\"type\":\"foundation.electrical.electrical\"}],\"Top\":[]}"
  ua1 : PMIOPort  Side=Left
  ua2 : PMIOPort  Port=2  Side=Right
  ub1 : PMIOPort  Port=3  Side=Left
  ub2 : PMIOPort  Port=4  Side=Right
  uc1 : PMIOPort  Port=5  Side=Left
  uc2 : PMIOPort  Port=6  Side=Right
  un1 : PMIOPort  Port=7  Side=Left
  un2 : PMIOPort  Port=8  Side=Right
  connections:
  uc2/RConn1 -- tr3/RConn1
  uc1/RConn1 -- tr3/LConn1
  ua1/RConn1 -- tr1/LConn1
  tr1/RConn1 -- ua2/RConn1
  ub2/RConn1 -- tr2/RConn1
  un1/RConn1 -- tr3/LConn2 -- tr2/LConn2 -- tr1/LConn2
  un2/RConn1 -- tr3/RConn2 -- tr2/RConn2 -- tr1/RConn2
  ub1/RConn1 -- tr2/LConn1

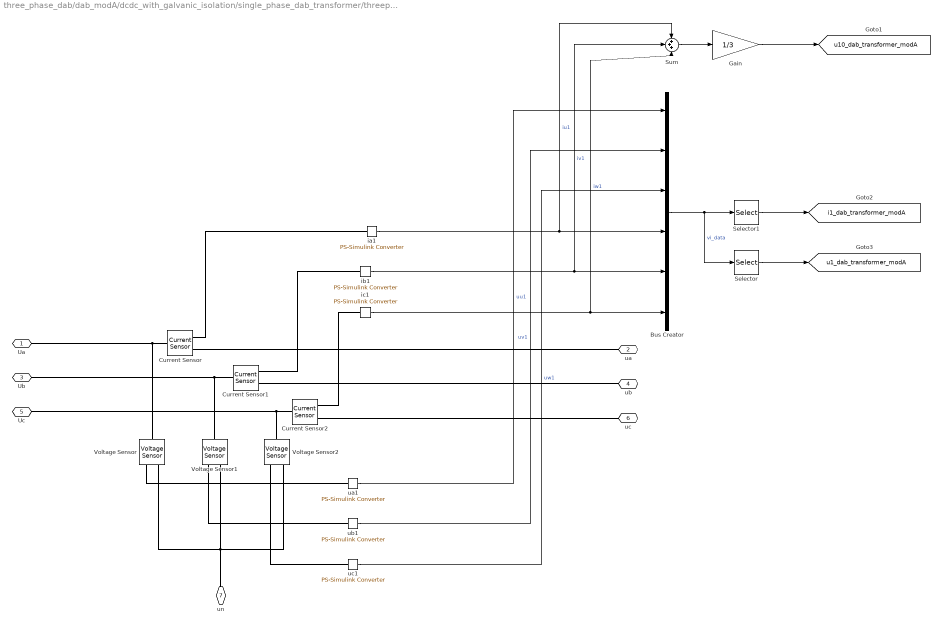
== system three_phase_dab/dab_modA/dcdc_with_galvanic_isolation/single_phase_dab_transformer/threephase_vi_measures_stack ==
  Bus Creator : BusCreator  Inputs=6
  Current Sensor : fl_lib/Electrical/Electrical Sensors/Current Sensor
  Current Sensor1 : fl_lib/Electrical/Electrical Sensors/Current Sensor
  Current Sensor2 : fl_lib/Electrical/Electrical Sensors/Current Sensor
  Gain : Gain  Gain=1/3
  Selector : Selector  InputPortWidth=6  IndexOptions=Index vector (dialog)  Indices=[1 2 3]  OutputSizes=1
  Selector1 : Selector  InputPortWidth=6  IndexOptions=Index vector (dialog)  Indices=[4 5 6]  OutputSizes=1
  Sum : Sum  Inputs=+++
  Voltage Sensor : fl_lib/Electrical/Electrical Sensors/Voltage Sensor
  Voltage Sensor1 : fl_lib/Electrical/Electrical Sensors/Voltage Sensor
  Voltage Sensor2 : fl_lib/Electrical/Electrical Sensors/Voltage Sensor
  ia1 : nesl_utility/PS-Simulink Converter  PhysicalDomain=network_engine_domain  SubClassName=ps_output  LeftPortType=input  RightPortType=output  PseudoPeriodic=off  Frequencies=[]  VectorFormat=1-D array  Unit=A  AffineConversion=off
  ib1 : nesl_utility/PS-Simulink Converter  PhysicalDomain=network_engine_domain  SubClassName=ps_output  LeftPortType=input  RightPortType=output  PseudoPeriodic=off  Frequencies=[]  VectorFormat=1-D array  Unit=A  AffineConversion=off
  ic1 : nesl_utility/PS-Simulink Converter  PhysicalDomain=network_engine_domain  SubClassName=ps_output  LeftPortType=input  RightPortType=output  PseudoPeriodic=off  Frequencies=[]  VectorFormat=1-D array  Unit=A  AffineConversion=off
  ua1 : nesl_utility/PS-Simulink Converter  PhysicalDomain=network_engine_domain  SubClassName=ps_output  LeftPortType=input  RightPortType=output  PseudoPeriodic=off  Frequencies=[]  VectorFormat=1-D array  Unit=V  AffineConversion=off
  ub1 : nesl_utility/PS-Simulink Converter  PhysicalDomain=network_engine_domain  SubClassName=ps_output  LeftPortType=input  RightPortType=output  PseudoPeriodic=off  Frequencies=[]  VectorFormat=1-D array  Unit=V  AffineConversion=off
  uc1 : nesl_utility/PS-Simulink Converter  PhysicalDomain=network_engine_domain  SubClassName=ps_output  LeftPortType=input  RightPortType=output  PseudoPeriodic=off  Frequencies=[]  VectorFormat=1-D array  Unit=V  AffineConversion=off
  Ua : PMIOPort  Side=Left
  ua : PMIOPort  Port=2  Side=Right
  Ub : PMIOPort  Port=3  Side=Left
  ub : PMIOPort  Port=4  Side=Right
  Uc : PMIOPort  Port=5  Side=Left
  uc : PMIOPort  Port=6  Side=Right
  un : PMIOPort  Port=7  Side=Right
  tag scope: i1_dab_transformer_modA=global, u10_dab_transformer_modA=global, u1_dab_transformer_modA=global
  wires:
  Bus Creator/1 -> Selector/1, Selector1/1  "vi_data"
  Selector/1 -> [u1_dab_transformer_modA]
  ib1/1 -> Sum/2, Bus Creator/5  "iv1"
  ia1/1 -> Sum/1, Bus Creator/4  "iu1"
  ic1/1 -> Bus Creator/6, Sum/3  "iw1"
  ua1/1 -> Bus Creator/1  "uu1"
  ub1/1 -> Bus Creator/2  "uv1"
  uc1/1 -> Bus Creator/3  "uw1"
  Selector1/1 -> [i1_dab_transformer_modA]
  Sum/1 -> Gain/1
  Gain/1 -> [u10_dab_transformer_modA]
  connections:
  Current Sensor1/LConn1 -- Ub/RConn1 -- Voltage Sensor1/LConn1
  Voltage Sensor/RConn2 -- un/RConn1 -- Voltage Sensor2/RConn2 -- Voltage Sensor1/RConn2
  Voltage Sensor/RConn1 -- ua1/LConn1
  Current Sensor/RConn2 -- ua/RConn1
  Voltage Sensor1/RConn1 -- ub1/LConn1
  Voltage Sensor2/LConn1 -- Uc/RConn1 -- Current Sensor2/LConn1
  Current Sensor/LConn1 -- Ua/RConn1 -- Voltage Sensor/LConn1
  Current Sensor1/RConn2 -- ub/RConn1
  Voltage Sensor2/RConn1 -- uc1/LConn1
  ib1/LConn1 -- Current Sensor1/RConn1
  ia1/LConn1 -- Current Sensor/RConn1
  ic1/LConn1 -- Current Sensor2/RConn1
  Current Sensor2/RConn2 -- uc/RConn1

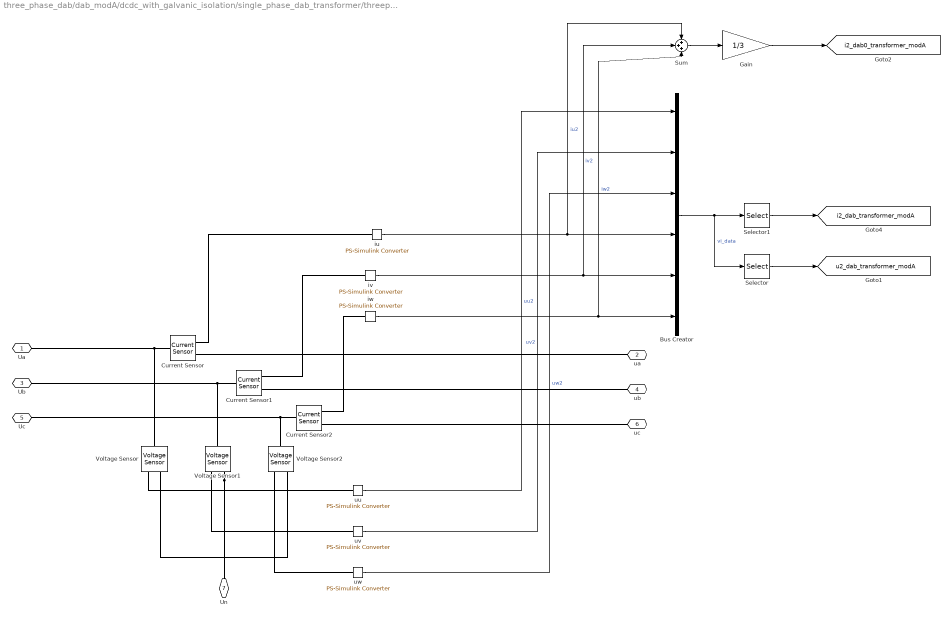
== system three_phase_dab/dab_modA/dcdc_with_galvanic_isolation/single_phase_dab_transformer/threephase_vi_measures_stack1 ==
  Bus Creator : BusCreator  Inputs=6
  Current Sensor : fl_lib/Electrical/Electrical Sensors/Current Sensor
  Current Sensor1 : fl_lib/Electrical/Electrical Sensors/Current Sensor
  Current Sensor2 : fl_lib/Electrical/Electrical Sensors/Current Sensor
  Gain : Gain  Gain=1/3
  Selector : Selector  InputPortWidth=6  IndexOptions=Index vector (dialog)  Indices=[1 2 3]  OutputSizes=1
  Selector1 : Selector  InputPortWidth=6  IndexOptions=Index vector (dialog)  Indices=[4 5 6]  OutputSizes=1
  Sum : Sum  Inputs=+++
  Voltage Sensor : fl_lib/Electrical/Electrical Sensors/Voltage Sensor
  Voltage Sensor1 : fl_lib/Electrical/Electrical Sensors/Voltage Sensor
  Voltage Sensor2 : fl_lib/Electrical/Electrical Sensors/Voltage Sensor
  iu : nesl_utility/PS-Simulink Converter  PhysicalDomain=network_engine_domain  SubClassName=ps_output  LeftPortType=input  RightPortType=output  PseudoPeriodic=off  Frequencies=[]  VectorFormat=1-D array  Unit=A  AffineConversion=off
  iv : nesl_utility/PS-Simulink Converter  PhysicalDomain=network_engine_domain  SubClassName=ps_output  LeftPortType=input  RightPortType=output  PseudoPeriodic=off  Frequencies=[]  VectorFormat=1-D array  Unit=A  AffineConversion=off
  iw : nesl_utility/PS-Simulink Converter  PhysicalDomain=network_engine_domain  SubClassName=ps_output  LeftPortType=input  RightPortType=output  PseudoPeriodic=off  Frequencies=[]  VectorFormat=1-D array  Unit=A  AffineConversion=off
  uu : nesl_utility/PS-Simulink Converter  PhysicalDomain=network_engine_domain  SubClassName=ps_output  LeftPortType=input  RightPortType=output  PseudoPeriodic=off  Frequencies=[]  VectorFormat=1-D array  Unit=V  AffineConversion=off
  uv : nesl_utility/PS-Simulink Converter  PhysicalDomain=network_engine_domain  SubClassName=ps_output  LeftPortType=input  RightPortType=output  PseudoPeriodic=off  Frequencies=[]  VectorFormat=1-D array  Unit=V  AffineConversion=off
  uw : nesl_utility/PS-Simulink Converter  PhysicalDomain=network_engine_domain  SubClassName=ps_output  LeftPortType=input  RightPortType=output  PseudoPeriodic=off  Frequencies=[]  VectorFormat=1-D array  Unit=V  AffineConversion=off
  Ua : PMIOPort  Side=Left
  ua : PMIOPort  Port=2  Side=Right
  Ub : PMIOPort  Port=3  Side=Left
  ub : PMIOPort  Port=4  Side=Right
  Uc : PMIOPort  Port=5  Side=Left
  uc : PMIOPort  Port=6  Side=Right
  Un : PMIOPort  Port=7  Side=Left
  tag scope: i2_dab0_transformer_modA=global, i2_dab_transformer_modA=global, u2_dab_transformer_modA=global
  wires:
  uu/1 -> Bus Creator/1  "uu2"
  Gain/1 -> [i2_dab0_transformer_modA]
  Sum/1 -> Gain/1
  Selector1/1 -> [i2_dab_transformer_modA]
  uw/1 -> Bus Creator/3  "uw2"
  uv/1 -> Bus Creator/2  "uv2"
  iw/1 -> Bus Creator/6, Sum/3  "iw2"
  iu/1 -> Bus Creator/4, Sum/1  "iu2"
  iv/1 -> Bus Creator/5, Sum/2  "iv2"
  Selector/1 -> [u2_dab_transformer_modA]
  Bus Creator/1 -> Selector1/1, Selector/1  "vi_data"
  connections:
  Current Sensor2/RConn2 -- uc/RConn1
  iw/LConn1 -- Current Sensor2/RConn1
  iu/LConn1 -- Current Sensor/RConn1
  iv/LConn1 -- Current Sensor1/RConn1
  Voltage Sensor2/RConn1 -- uw/LConn1
  Current Sensor1/RConn2 -- ub/RConn1
  Voltage Sensor/LConn1 -- Ua/RConn1 -- Current Sensor/LConn1
  Current Sensor2/LConn1 -- Uc/RConn1 -- Voltage Sensor2/LConn1
  Voltage Sensor1/RConn1 -- uv/LConn1
  Current Sensor/RConn2 -- ua/RConn1
  Voltage Sensor/RConn1 -- uu/LConn1
  Voltage Sensor1/RConn2 -- Un/RConn1 -- Voltage Sensor2/RConn2 -- Voltage Sensor/RConn2
  Voltage Sensor1/LConn1 -- Ub/RConn1 -- Current Sensor1/LConn1

== system three_phase_dab/dab_modA/dcdc_with_galvanic_isolation/three_phase_inverter_1/dclink_1 ==
  CFi_dc1 : fl_lib/Electrical/Electrical Elements/Capacitor  c=CFi_dc1 F  r=RCFi_dc1_internal Ohm  g=0 1/Ohm  i_specify=off  i_priority=None  i=0 A  i_nominal_specify=off  i_nominal_value=1  i_nominal_unit=A  v_specify=off  v_priority=None  v=0 V  v_nominal_specify=off  v_nominal_value=1  v_nominal_unit=V  vc_specify=off  vc_priority=High  vc=0 V  vc_nominal_specify=off  vc_nominal_value=1  vc_nominal_unit=V
  Current Sensor : fl_lib/Electrical/Electrical Sensors/Current Sensor
  PS-Simulink Converter1 : nesl_utility/PS-Simulink Converter  PhysicalDomain=network_engine_domain  SubClassName=ps_output  LeftPortType=input  RightPortType=output  PseudoPeriodic=off  Frequencies=[]  VectorFormat=1-D array  Unit=A  AffineConversion=on
  PS-Simulink Converter4 : nesl_utility/PS-Simulink Converter  PhysicalDomain=network_engine_domain  SubClassName=ps_output  LeftPortType=input  RightPortType=output  PseudoPeriodic=off  Frequencies=[]  VectorFormat=1-D array  Unit=V  AffineConversion=on
  Voltage Sensor : fl_lib/Electrical/Electrical Sensors/Voltage Sensor
  udc(+) : PMIOPort  Side=Left
  Udc(+) : PMIOPort  Port=2  Side=Right
  udc(-) : PMIOPort  Port=3  Side=Left
  Udc(-) : PMIOPort  Port=4  Side=Right
  tag scope: CFi_dc_current=global, dab_voltage_input_modA=global
  wires:
  PS-Simulink Converter4/1 -> [dab_voltage_input_modA]  "dab_voltage_input_modA"
  PS-Simulink Converter1/1 -> [CFi_dc_current]  "CFi_dc_current"
  connections:
  Current Sensor/RConn1 -- PS-Simulink Converter1/LConn1
  PS-Simulink Converter4/LConn1 -- Voltage Sensor/RConn1
  Current Sensor/LConn1 -- CFi_dc1/RConn1
  Voltage Sensor/RConn2 -- Current Sensor/RConn2 -- Udc(-)/RConn1 -- udc(-)/RConn1
  CFi_dc1/LConn1 -- Udc(+)/RConn1 -- udc(+)/RConn1 -- Voltage Sensor/LConn1

== system three_phase_dab/dab_modA/dcdc_with_galvanic_isolation/three_phase_inverter_1/three_phase_inverter_1 ==
  gate_commands : Inport
  three_phase_inverter_ideal_switch_based_model : three_phase_inverter_ideal_switch_based_model/three phase inverter ideal switch based model  Commented=on  Ron_ideal_switch=Rds_on  Vth=Vth  Vgamma=Vdon_diode  Rdon_diode=Rdon_diode  Csnubber=Csnubber  Rsnubber=Rsnubber
  three_phase_inverter_mosfet_based_with_thermal_model : three_phase_inverter_mosfet_based_with_thermal_model/three phase inverter mosfet based with thermal model  mass_heatsink=0.2  specific_heat=cp_al  rth_mosfet_HA=Rth_mosfet_HA  rth_mosfet_JH=Rth_mosfet_JH  Rds_on=Rds_on  Vth=Vth  Eon=Eon  Eoff=Eoff  Voff_sw_loss=Voff_sw_losses  Ion_sw_loss=Ion_sw_losses  Vdon_diode=Vdon_diode  Rdon_diode=Rdon_diode  JunctionTermalMass=JunctionTermalMass  Tambient=Tambient  DThs_init=DThs_init
  udc(+) : PMIOPort  Side=Left
  u : PMIOPort  Port=2  Side=Right
  v : PMIOPort  Port=3  Side=Right
  udc(-) : PMIOPort  Port=4  Side=Left
  w : PMIOPort  Port=5  Side=Right
  tag scope: inverter_1_dab_devices_modA=global
  wires:
  gate_commands/1 -> three_phase_inverter_ideal_switch_based_model/1, three_phase_inverter_mosfet_based_with_thermal_model/1
  three_phase_inverter_mosfet_based_with_thermal_model/1 -> [inverter_1_dab_devices_modA]
  connections:
  u/RConn1 -- three_phase_inverter_ideal_switch_based_model/RConn1 -- three_phase_inverter_mosfet_based_with_thermal_model/RConn1
  v/RConn1 -- three_phase_inverter_ideal_switch_based_model/RConn2 -- three_phase_inverter_mosfet_based_with_thermal_model/RConn2
  udc(-)/RConn1 -- three_phase_inverter_ideal_switch_based_model/LConn2 -- three_phase_inverter_mosfet_based_with_thermal_model/LConn2
  w/RConn1 -- three_phase_inverter_ideal_switch_based_model/RConn3 -- three_phase_inverter_mosfet_based_with_thermal_model/RConn3
  udc(+)/RConn1 -- three_phase_inverter_ideal_switch_based_model/LConn1 -- three_phase_inverter_mosfet_based_with_thermal_model/LConn1
